simulink model "ToVineetha2023bLasttryf"  (R2023b)
settings: Solver=ode45  StartTime=0.0  StopTime=0.7  MaxStep=5*10^-6  RelTol=1e-3
libraries: spsdq0toabcLib x2
settings Model: Creator=villiamp  LastModifiedBy=villiamp
settings RTWCC: GPUComputeCapability=5.0

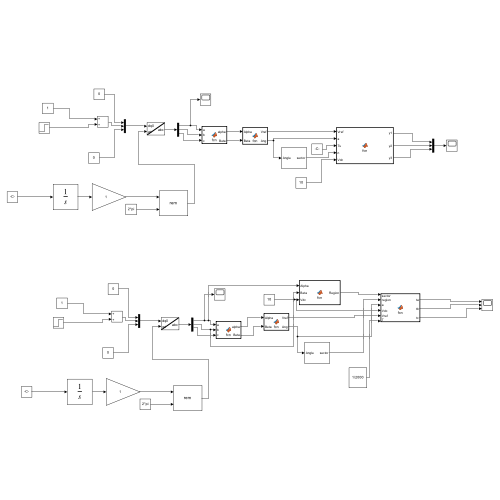
[thumbnail: Simulink's stored preview of the top-level diagram]
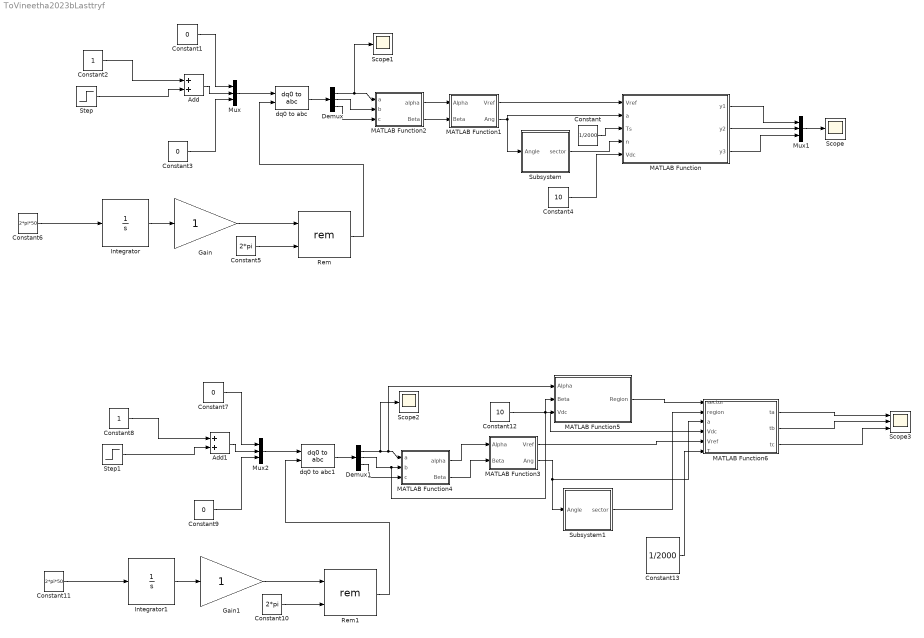
== system ToVineetha2023bLasttryf ==
  Add : Sum
  Add1 : Sum
  Constant : Constant  Value=1/2000
  Constant{1,3,7,9} (4 alike) : Constant  Value=0
  Constant10 : Constant  Value=2*pi
  Constant11 : Constant  Value=2*pi*50
  Constant12 : Constant  Value=10
  Constant13 : Constant  Value=1/2000
  Constant2 : Constant
  Constant4 : Constant  Value=10
  Constant5 : Constant  Value=2*pi
  Constant6 : Constant  Value=2*pi*50
  Constant8 : Constant
  Demux : Demux  Outputs=3
  Demux1 : Demux  Outputs=3
  Gain : Gain
  Gain1 : Gain
  Integrator : Integrator
  Integrator1 : Integrator
  MATLAB Function : MATLAB Function  TreatAsAtomicUnit=on
  MATLAB Function1 : MATLAB Function  TreatAsAtomicUnit=on
  MATLAB Function2 : MATLAB Function  TreatAsAtomicUnit=on
  MATLAB Function3 : MATLAB Function  TreatAsAtomicUnit=on
  MATLAB Function4 : MATLAB Function  TreatAsAtomicUnit=on
  MATLAB Function5 : MATLAB Function  TreatAsAtomicUnit=on
  MATLAB Function6 : MATLAB Function  TreatAsAtomicUnit=on
  Mux : Mux  Inputs=3
  Mux1 : Mux  Inputs=3
  Mux2 : Mux  Inputs=3
  Rem : Math  Operator=rem
  Rem1 : Math  Operator=rem
  Scope : Scope
  Scope1 : Scope
  Scope2 : Scope
  Scope3 : Scope  NumInputPorts=3
  Step : Step  Time=0.5  After=4  SampleTime=0
  Step1 : Step  Time=0.5  After=4  SampleTime=0
  Subsystem : Subsystem
  Subsystem1 : Subsystem
  dq0 to abc : spsdq0toabcLib/dq0 to abc  Alignment=90 degrees behind phase A axis
  dq0 to abc1 : spsdq0toabcLib/dq0 to abc  Alignment=90 degrees behind phase A axis
  wires:
  Constant/1 -> MATLAB Function/3(Ts)
  Subsystem/1(sector) -> MATLAB Function/4(n)
  MATLAB Function/3(y3) -> Mux1/3
  Mux1/1 -> Scope/1
  MATLAB Function2/1(alpha) -> MATLAB Function1/1(Alpha)
  MATLAB Function2/2(Beta) -> MATLAB Function1/2(Beta)
  MATLAB Function1/1(Vref) -> MATLAB Function/1(Vref)
  MATLAB Function1/2(Ang) -> Subsystem/1(Angle), MATLAB Function/2(a)
  Mux/1 -> dq0 to abc/1
  Constant1/1 -> Mux/1
  Add/1 -> Mux/2
  Demux/1 -> Scope1/1, MATLAB Function2/1(a)
  dq0 to abc/1 -> Demux/1
  Demux/2 -> MATLAB Function2/2(b)
  Demux/3 -> MATLAB Function2/3(c)
  Step/1 -> Add/2
  Constant2/1 -> Add/1
  Constant3/1 -> Mux/3
  Constant4/1 -> MATLAB Function/5(Vdc)
  Constant5/1 -> Rem/2
  Gain/1 -> Rem/1
  Integrator/1 -> Gain/1
  Constant6/1 -> Integrator/1
  Rem/1 -> dq0 to abc/2
  MATLAB Function/2(y2) -> Mux1/2
  MATLAB Function/1(y1) -> Mux1/1
  Integrator1/1 -> Gain1/1
  Gain1/1 -> Rem1/1
  Constant10/1 -> Rem1/2
  Constant11/1 -> Integrator1/1
  Add1/1 -> Mux2/2
  dq0 to abc1/1 -> Demux1/1
  Constant7/1 -> Mux2/1
  Rem1/1 -> dq0 to abc1/2
  Constant8/1 -> Add1/1
  Constant9/1 -> Mux2/3
  Demux1/3 -> MATLAB Function4/3(c)
  Demux1/1 -> Scope2/1, MATLAB Function5/1(Alpha), MATLAB Function4/1(a)
  Mux2/1 -> dq0 to abc1/1
  Step1/1 -> Add1/2
  MATLAB Function3/2(Ang) -> Subsystem1/1(Angle), MATLAB Function6/3(a)
  MATLAB Function4/1(alpha) -> MATLAB Function3/1(Alpha)
  MATLAB Function4/2(Beta) -> MATLAB Function3/2(Beta)
  Demux1/2 -> MATLAB Function5/2(Beta), MATLAB Function4/2(b)
  Constant12/1 -> MATLAB Function6/4(Vdc), MATLAB Function5/3(Vdc)
  MATLAB Function5/1(Region) -> MATLAB Function6/1(sector)
  Subsystem1/1(sector) -> MATLAB Function6/2(region)
  MATLAB Function3/1(Vref) -> MATLAB Function6/5(Vref)
  Constant13/1 -> MATLAB Function6/6(T)
  MATLAB Function6/1(ta) -> Scope3/1
  MATLAB Function6/2(tb) -> Scope3/2
  MATLAB Function6/3(tc) -> Scope3/3

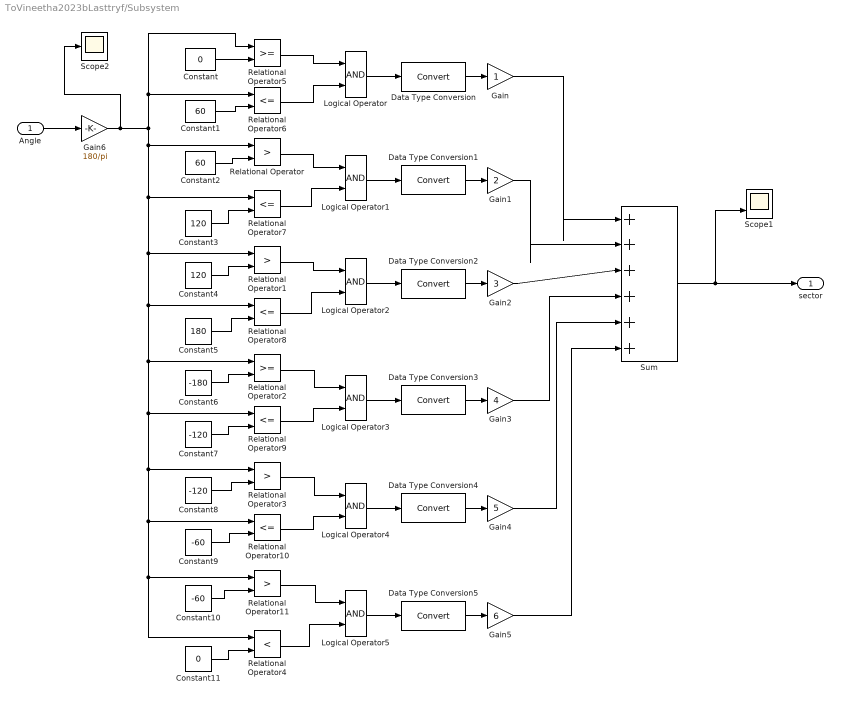
== system ToVineetha2023bLasttryf/Subsystem ==
  Angle : Inport
  Constant : Constant  Value=0
  Constant1 : Constant  Value=60
  Constant10 : Constant  Value=-60
  Constant11 : Constant  Value=0
  Constant2 : Constant  Value=60
  Constant3 : Constant  Value=120
  Constant4 : Constant  Value=120
  Constant5 : Constant  Value=180
  Constant6 : Constant  Value=-180
  Constant7 : Constant  Value=-120
  Constant8 : Constant  Value=-120
  Constant9 : Constant  Value=-60
  Data Type Conversion{,1..5} (6 alike) : DataTypeConversion  SaturateOnIntegerOverflow=off  RndMeth=Floor
  Gain : Gain
  Gain1 : Gain  Gain=2
  Gain2 : Gain  Gain=3
  Gain3 : Gain  Gain=4
  Gain4 : Gain  Gain=5
  Gain5 : Gain  Gain=6
  Gain6 : Gain  Gain=180/pi
  Logical Operator{,1..5} (6 alike) : Logic  AllPortsSameDT=off  OutDataTypeStr=boolean
  Relational Operator{,1,3,11} (4 alike) : RelationalOperator  Operator=>  OutDataTypeStr=boolean  InputSameDT=off
  Relational Operator{6..10} (5 alike) : RelationalOperator  Operator=<=  OutDataTypeStr=boolean  InputSameDT=off
  Relational Operator2 : RelationalOperator  OutDataTypeStr=boolean  InputSameDT=off
  Relational Operator4 : RelationalOperator  Operator=<  OutDataTypeStr=boolean  InputSameDT=off
  Relational Operator5 : RelationalOperator  OutDataTypeStr=boolean  InputSameDT=off
  Scope1 : Scope  NumInputPorts=2
  Scope2 : Scope
  Sum : Sum  Inputs=|++++++
  sector : Outport
  wires:
  Relational Operator11/1 -> Logical Operator5/1
  Gain6/1 -> Scope2/1, Relational Operator5/1, Relational Operator6/1, Relational Operator4/1, Relational Operator11/1, Relational Operator10/1, Relational Operator3/1, Relational Operator9/1, Relational Operator2/1, Relational Operator8/1, Relational Operator1/1, Relational Operator7/1, Relational Operator/1
  Relational Operator6/1 -> Logical Operator/2
  Constant9/1 -> Relational Operator10/2
  Logical Operator5/1 -> Data Type Conversion5/1
  Sum/1 -> sector/1, Scope1/2
  Constant1/1 -> Relational Operator6/2
  Relational Operator4/1 -> Logical Operator5/2
  Constant3/1 -> Relational Operator7/2
  Data Type Conversion3/1 -> Gain3/1
  Data Type Conversion/1 -> Gain/1
  Constant/1 -> Relational Operator5/2
  Logical Operator3/1 -> Data Type Conversion3/1
  Data Type Conversion5/1 -> Gain5/1
  Logical Operator1/1 -> Data Type Conversion1/1
  Constant8/1 -> Relational Operator3/2
  Data Type Conversion4/1 -> Gain4/1
  Gain1/1 -> Sum/2
  Constant5/1 -> Relational Operator8/2
  Relational Operator7/1 -> Logical Operator1/2
  Constant6/1 -> Relational Operator2/2
  Relational Operator9/1 -> Logical Operator3/2
  Constant10/1 -> Relational Operator11/2
  Relational Operator5/1 -> Logical Operator/1
  Logical Operator4/1 -> Data Type Conversion4/1
  Logical Operator/1 -> Data Type Conversion/1
  Data Type Conversion1/1 -> Gain1/1
  Constant2/1 -> Relational Operator/2
  Relational Operator1/1 -> Logical Operator2/1
  Relational Operator10/1 -> Logical Operator4/2
  Relational Operator8/1 -> Logical Operator2/2
  Constant7/1 -> Relational Operator9/2
  Angle/1 -> Gain6/1
  Data Type Conversion2/1 -> Gain2/1
  Logical Operator2/1 -> Data Type Conversion2/1
  Gain5/1 -> Sum/6
  Relational Operator3/1 -> Logical Operator4/1
  Gain2/1 -> Sum/3
  Gain4/1 -> Sum/5
  Gain/1 -> Sum/1
  Gain3/1 -> Sum/4
  Constant11/1 -> Relational Operator4/2
  Relational Operator2/1 -> Logical Operator3/1
  Relational Operator/1 -> Logical Operator1/1
  Constant4/1 -> Relational Operator1/2

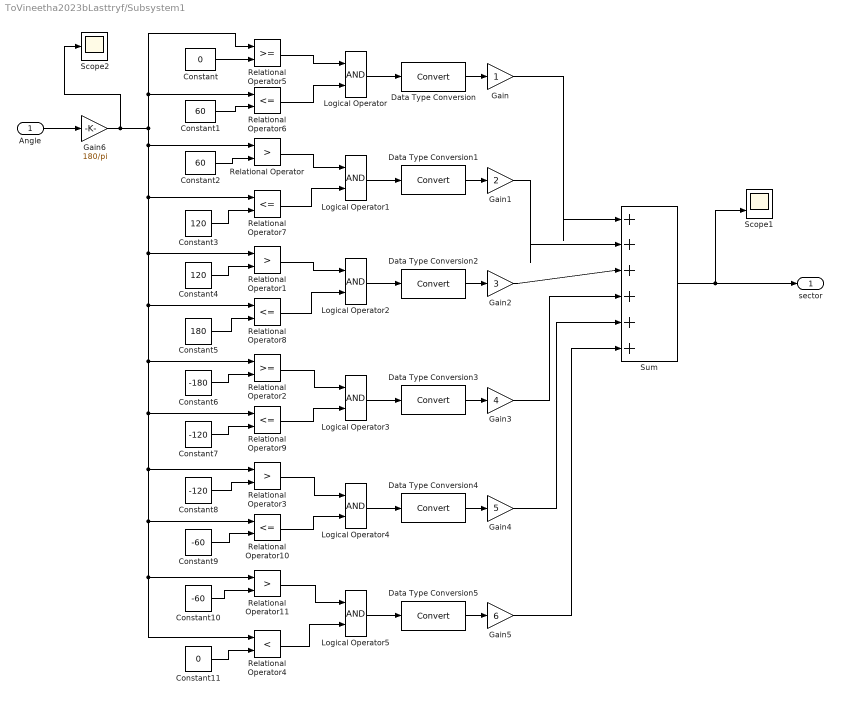
== system ToVineetha2023bLasttryf/Subsystem1 ==
  Angle : Inport
  Constant : Constant  Value=0
  Constant1 : Constant  Value=60
  Constant10 : Constant  Value=-60
  Constant11 : Constant  Value=0
  Constant2 : Constant  Value=60
  Constant3 : Constant  Value=120
  Constant4 : Constant  Value=120
  Constant5 : Constant  Value=180
  Constant6 : Constant  Value=-180
  Constant7 : Constant  Value=-120
  Constant8 : Constant  Value=-120
  Constant9 : Constant  Value=-60
  Data Type Conversion{,1..5} (6 alike) : DataTypeConversion  SaturateOnIntegerOverflow=off  RndMeth=Floor
  Gain : Gain
  Gain1 : Gain  Gain=2
  Gain2 : Gain  Gain=3
  Gain3 : Gain  Gain=4
  Gain4 : Gain  Gain=5
  Gain5 : Gain  Gain=6
  Gain6 : Gain  Gain=180/pi
  Logical Operator{,1..5} (6 alike) : Logic  AllPortsSameDT=off  OutDataTypeStr=boolean
  Relational Operator{,1,3,11} (4 alike) : RelationalOperator  Operator=>  OutDataTypeStr=boolean  InputSameDT=off
  Relational Operator{6..10} (5 alike) : RelationalOperator  Operator=<=  OutDataTypeStr=boolean  InputSameDT=off
  Relational Operator2 : RelationalOperator  OutDataTypeStr=boolean  InputSameDT=off
  Relational Operator4 : RelationalOperator  Operator=<  OutDataTypeStr=boolean  InputSameDT=off
  Relational Operator5 : RelationalOperator  OutDataTypeStr=boolean  InputSameDT=off
  Scope1 : Scope  NumInputPorts=2
  Scope2 : Scope
  Sum : Sum  Inputs=|++++++
  sector : Outport
  wires:
  Relational Operator11/1 -> Logical Operator5/1
  Gain6/1 -> Scope2/1, Relational Operator5/1, Relational Operator6/1, Relational Operator4/1, Relational Operator11/1, Relational Operator10/1, Relational Operator3/1, Relational Operator9/1, Relational Operator2/1, Relational Operator8/1, Relational Operator1/1, Relational Operator7/1, Relational Operator/1
  Relational Operator6/1 -> Logical Operator/2
  Constant9/1 -> Relational Operator10/2
  Logical Operator5/1 -> Data Type Conversion5/1
  Sum/1 -> sector/1, Scope1/2
  Constant1/1 -> Relational Operator6/2
  Relational Operator4/1 -> Logical Operator5/2
  Constant3/1 -> Relational Operator7/2
  Data Type Conversion3/1 -> Gain3/1
  Data Type Conversion/1 -> Gain/1
  Constant/1 -> Relational Operator5/2
  Logical Operator3/1 -> Data Type Conversion3/1
  Data Type Conversion5/1 -> Gain5/1
  Logical Operator1/1 -> Data Type Conversion1/1
  Constant8/1 -> Relational Operator3/2
  Data Type Conversion4/1 -> Gain4/1
  Gain1/1 -> Sum/2
  Constant5/1 -> Relational Operator8/2
  Relational Operator7/1 -> Logical Operator1/2
  Constant6/1 -> Relational Operator2/2
  Relational Operator9/1 -> Logical Operator3/2
  Constant10/1 -> Relational Operator11/2
  Relational Operator5/1 -> Logical Operator/1
  Logical Operator4/1 -> Data Type Conversion4/1
  Logical Operator/1 -> Data Type Conversion/1
  Data Type Conversion1/1 -> Gain1/1
  Constant2/1 -> Relational Operator/2
  Relational Operator1/1 -> Logical Operator2/1
  Relational Operator10/1 -> Logical Operator4/2
  Relational Operator8/1 -> Logical Operator2/2
  Constant7/1 -> Relational Operator9/2
  Angle/1 -> Gain6/1
  Data Type Conversion2/1 -> Gain2/1
  Logical Operator2/1 -> Data Type Conversion2/1
  Gain5/1 -> Sum/6
  Relational Operator3/1 -> Logical Operator4/1
  Gain2/1 -> Sum/3
  Gain4/1 -> Sum/5
  Gain/1 -> Sum/1
  Gain3/1 -> Sum/4
  Constant11/1 -> Relational Operator4/2
  Relational Operator2/1 -> Logical Operator3/1
  Relational Operator/1 -> Logical Operator1/1
  Constant4/1 -> Relational Operator1/2

== matlab function ToVineetha2023bLasttryf/MATLAB Function1 ==
  data: Vref output; Alpha input; Ang output; Beta input
function [Vref,Ang] = fcn(Alpha,Beta)
Ang=atan2(Beta,Alpha);
Vref=sqrt(Alpha^2+Beta^2);

== matlab function ToVineetha2023bLasttryf/MATLAB Function ==
  data: Vref input; a input; y1 output; Ts input; n input; y2 output; y3 output; Vdc input
function [y1,y2,y3] = fcn(Vref,a,Ts,n,Vdc)
y1=0;
y2=0;
y3=0;
m=Ts*sqrt(3)/2*Vref/Vdc/2;
T1=m*sin(n*pi/3-a);
T2=m*sin(a-(n-1)/3*pi);
T0=Ts-T1-T2;
if n==1
y1=T0/2+T1+T2;
y2=T2+T0/2;
y3=T0/2;
end
if n==2
y1=T1+T0/2;
y2=T1+T2+T0/2;
y3=T0/2;
end 
if n==3
y1=T0/2;
y2=T1+T2+T0/2;
y3=T2+T0/2;
end 
if n==4
y1=T0/2;
y2=T1+T0/2;
y3=T1+T2+T0/2;
end 
if n==5
y1=T2+T0/2; 
y2=T0/2;
y3=T1+T2+T0/2;
end
if n==6
y1=T0/2+T2+T1;
y2=T0/2;
y3=T1+T0/2;
end

== matlab function ToVineetha2023bLasttryf/MATLAB Function2 ==
  data: a input; alpha output; b input; c input; Beta output
function [alpha,Beta] = fcn(a,b,c)


% Clark transformation matrix
Clark= (2/3) * [1, -0.5, -0.5; 0, sqrt(3)/2, -sqrt(3)/2];
Result=Clark*[a,b,c]';
alpha=Result(1);
Beta=Result(2);

== matlab function ToVineetha2023bLasttryf/MATLAB Function3 ==
  data: Vref output; Alpha input; Ang output; Beta input
function [Vref,Ang] = fcn(Alpha,Beta)
Ang=atan2(Beta,Alpha);
Vref=sqrt(Alpha^2+Beta^2);

== matlab function ToVineetha2023bLasttryf/MATLAB Function4 ==
  data: a input; alpha output; b input; c input; Beta output
function [alpha,Beta] = fcn(a,b,c)


% Clark transformation matrix
Clark= (2/3) * [1, -0.5, -0.5; 0, sqrt(3)/2, -sqrt(3)/2];
Result=Clark*[a,b,c]';
alpha=Result(1);
Beta=Result(2);

== matlab function ToVineetha2023bLasttryf/MATLAB Function5 ==
  data: Region output; Alpha input; Beta input; Vdc input
function Region  = fcn(Alpha,Beta,Vdc)
Region=0;
R1=Alpha+sqrt(3)/3*Beta-Vdc/3;
R2=Alpha-sqrt(3)/3*Beta-Vdc/3;
R3=Alpha-sqrt(3)/6*Vdc;

if R1<0
    Region=1;
elseif R2>0
    Region=3;
elseif R3<0
    Region=4;
else 
    Region=2;
end

== matlab function ToVineetha2023bLasttryf/MATLAB Function6 ==
  data: sector input; ta output; region input; a input; Vdc input; Vref input; T input; tb output; tc output
function [ta,tb,tc] = fcn(sector,region,a,Vdc,Vref,T)
V=Vref/(4/3*Vdc);
q=2*V/sqrt(3);
ta=0;
tb=0;
tc=0;
%SECTOR1
if sector==1 && region==1
    ta=q*T*sin(pi/3-a);
    tb=T/2*(1-2*q*sin(a+pi/3));
    tc=a*T*sin(a);
end 
if sector==1 && region==2
    ta=T*(1+q*sin(a-pi/3));
    tb=-q*T*sin(a);
    tc=-T/2*(2*q*sin(a)-1);
end 
if sector==1 && region==3
    ta=T/2*(1-2*q*sin(a));
    tb=T/2*(2*q*sin(a+pi/3)-2);
    tc=T/2*(1+2*q*sin(a-pi/3));
end 
if sector==1 && region==4
    ta=T/2*(2*q*sin(a)-1);
    tb=q*T*sin(pi/3-a);
    tc=T*(1-2*q*sin(a+pi/3));
end 
%sector2
%%%%%%%%%%%%%%%%%%%%%%%%%%%%%%%%%%%%%%%%%%%%
if sector==2 && region==1
    ta=q*T*sin(pi/3-a);
    tb=T/2*(1-2*q*sin(a+pi/3));
    tc=q*T*sin(a);
end 
if sector==2 && region==2
    ta=T/2*(2*q*sin(pi/3+a)-1);
    tb=-q*T*sin(pi/3-a);
    tc=T*(1-q*sin(a));
end 
if sector==2 && region==3
    ta=T/2*(1-2*q*sin(a+pi/3));
    tb=T/2*(2*q*sin(a)-1);
    tc=T/2*(2*q*sin(pi/3-a)+1);
end 
if sector==2 && region==4
    ta=T*(1-q*sin(a));
    tb=q*T*sin(pi/3+a);
    tc=T/2*(2*q*sin(a-pi/3)-1);
end 
%sector3
%%%%%%%%%%%%%%%%%%%%%%%%%%%%%%%%%%%%%%%%%%%%
if sector==3 && region==1
    ta=q*T*sin(a);
    tb=T/2*(1-2*q*sin(a-pi/3));
    tc=-q*T*sin(a+pi/3);
end 
if sector==3 && region==2
    ta=T*(1-q*sin(a-pi/3));
    tb=-q*T*sin(pi/3+a);
    tc=-T/2*(2*q*sin(a)-1);
end 
if sector==3 && region==3
    ta=T/2*(2*q*sin(a+pi/3)+1);
    tb=-T/2*(1+2*q*sin(pi/3-a));
    tc=T/2*(1-2*q*sin(a));
end 
if sector==3 && region==4
    ta=-T/2*(1-q*sin(a));
    tb=q*T*sin(pi/3+a);
    tc=T/2*(2*q*sin(a-pi/3)-1);
end 
%sector4
%%%%%%%%%%%%%%%%%%%%%%%%%%%%%%%%%%%%%%%%%%%%
if sector==4 && region==1
    ta=-q*T*sin(a);
    tb=T/2*(1+2*q*sin(a+pi/3));
    tc=q*T*sin(a-pi/3);
end 
if sector==4 && region==2
    ta=T/2*(q*2*sin(a-pi/3)-1);
    tb=-q*T*sin(a);
    tc=T*(1+q*sin(a+pi/3));
end 
if sector==4 && region==3
    ta=T/2*(2*q*sin(a-pi/3)-1);
    tb=-T/2*(1+2*q*sin(a+pi/3));
    tc=T/2*(1+2*q*sin(a));
end 
if sector==4 && region==4
    ta=-T/2*(1+q*sin(a+pi/3));
    tb=q*T*sin(a);
    tc=T*(1+q*sin(pi/3-a));
end 
%sector5
%%%%%%%%%%%%%%%%%%%%%%%%%%%%%%%%%%%%%%%%%%%%
if sector==5 && region==1
    ta=-q*T*sin(a+pi/3);
    tb=T/2*(1+2*q*sin(a));
    tc=q*T*sin(pi/3-a);
end 
if sector==5 && region==2
    ta=T*(1+q*sin(a));
    tb=q*T*sin(pi/3-a);
    tc=T/2*(2*q*sin(a+pi/3)+1);
end 
if sector==5 && region==3
    ta=T/2*(2*q*sin(a-pi/3)+1);
    tb=-T/2*(2*q*sin(a)+1);
    tc=T/2*(2*q*sin(a+pi/3)+1);
end 
if sector==5 && region==4
    ta=T/2*(2*q*sin(pi/3-a)-1);
    tb=-q*T*sin(a+pi/3);
    tc=T*(1+q*sin(a));
end 
%sector6
%%%%%%%%%%%%%%%%%%%%%%%%%%%%%%%%%%%%%%%%%%%%
if sector==6 && region==1
    ta=q*T*sin(a+pi/3);
    tb=T/2*(1+2*q*sin(a-pi/3));
    tc=-q*T*sin(a);
end 
if sector==6 && region==2
    ta=-T*(1+2*q*sin(a));
    tb=q*T*sin(a+pi/3);
    tc=T/2*(q*sin(a-pi/3)+1);
end 
if sector==6 && region==3
    ta=T/2*(2*q*sin(a)+1);
    tb=T/2*(1-2*q*sin(a+pi/3));
    tc=T/2*(2*q*sin(pi/3-a)-1);
end 
if sector==6 && region==4
    ta=T*(1+q*sin(a-pi/3));
    tb=-q*T*sin(a);
    tc=-T/2*(2*q*sin(a+pi/3)-1);
end
